simulink model "speedgoat deneme"  (R2015b)
settings: Solver=FixedStepDiscrete  StartTime=0.0  StopTime=inf  RelTol=1e-3
libraries: speedgoatlib_IO102 x4, speedgoatlib_fpga x3, slrtlib x2, simulink x1
settings Model: Creator=PowerLab  LastModifiedBy=PowerLab
settings SolverCC: EnableConcurrentExecution=on
settings OptimizationCC: BlockReduction=off  OptimizeBlockIOStorage=off  BufferReuse=off  GlobalBufferReuse=off  ExpressionFolding=off  LocalBlockOutputs=off
settings HardwareCC: ProdBitPerPointer=32  ProdLargestAtomicFloat=None  ProdWordSize=32  ProdLongLongMode=on  ProdHWDeviceType=Generic->32-bit x86 compatible
settings RTWCC: SystemTargetFile=slrt.tlc  TemplateMakefile=slrt_default_tmf  Description=Simulink Real-Time  RTWCompilerOptimization=on
settings SimulinkRealTimeCC: xPCisModelTimeout=off  xPCModelTimeoutSecs=20

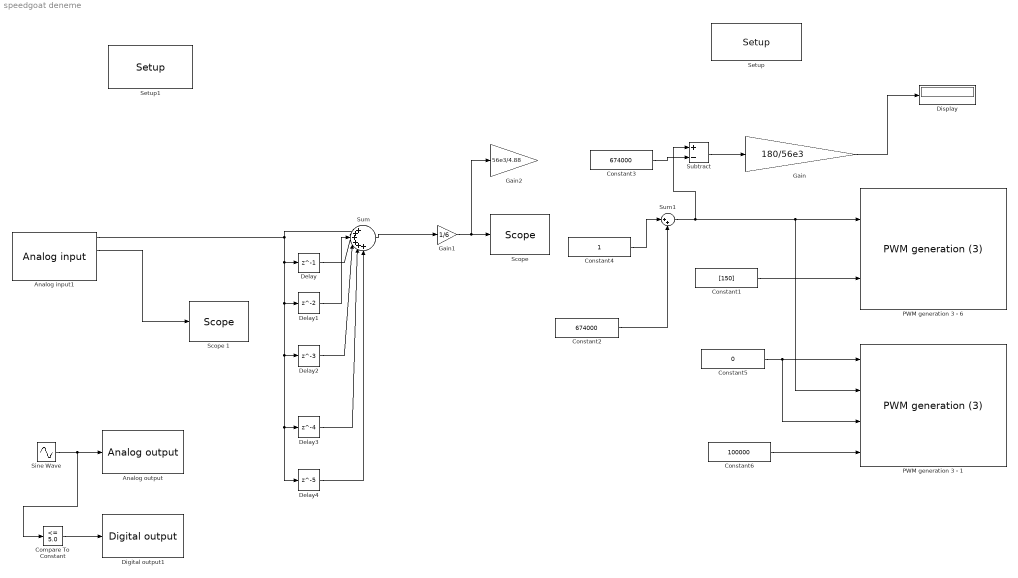
== system speedgoat deneme ==
  Analog input1 : speedgoatlib_IO102/Analog input  id=1  channels=[1,2,3,4]  range=1  high_voltage=off  adCoupling=1  ts=0.001  pciSlot=-1
  Analog output : speedgoatlib_IO102/Analog output  id=1  channels=1  range=1  ts=0.0001  pciSlot=-1
  Compare To Constant : simulink/Logic and Bit Operations/Compare To Constant  relop=<=  const=5.0  OutDataTypeStr=boolean
  Constant1 : Constant  Value=[150]  VectorParams1D=off  OutDataTypeStr=Inherit: Inherit via back propagation
  Constant2 : Constant  Value=674000  VectorParams1D=off  OutDataTypeStr=Inherit: Inherit via back propagation
  Constant3 : Constant  Value=674000  VectorParams1D=off  OutDataTypeStr=Inherit: Inherit via back propagation
  Constant4 : Constant  VectorParams1D=off  OutDataTypeStr=Inherit: Inherit via back propagation
  Constant5 : Constant  Value=0  VectorParams1D=off  OutDataTypeStr=Inherit: Inherit via back propagation
  Constant6 : Constant  Value=100000  VectorParams1D=off  OutDataTypeStr=Inherit: Inherit via back propagation
  Delay : Delay  DelayLength=1
  Delay1 : Delay
  Delay2 : Delay  DelayLength=3
  Delay3 : Delay  DelayLength=4
  Delay4 : Delay  DelayLength=5
  Digital output1 : speedgoatlib_IO102/Digital output  id=1  channels=1  ts=0.001  pciSlot=-1
  Display : Display
  Gain : Gain  Gain=180/56e3
  Gain1 : Gain  Gain=1/6
  Gain2 : Gain  Gain=56e3/4.88
  PWM generation 3 - 1 : speedgoatlib_fpga/PWM/PWM generation (3)  id=1  chan=[1]  board=IO316  ts=0.001  pciSlot=-1  symmetric=Asymmetric - On and Off are freely configurable  period=[1500000]  invertA=High between AOn and AOff  invertB=Low between BOn and BOff  invertC=High during PWM strobe  triggerSource=Period starts  triggerPulseLength=[255]  protection=Disabled: A and B can be high at the same moment  update=At period starts  idleA=Low when PWM generation is halted  idleB=Low when PWM generation is halted
  PWM generation 3 - 6 : speedgoatlib_fpga/PWM/PWM generation (3)  id=1  chan=[3]  board=IO316  ts=0.001  pciSlot=-1  symmetric=Symmetric - PWM generation is centered around half the period  period=[1500000]  invertA=High between AOn and AOff  invertB=High between BOn and BOff  invertC=High during PWM strobe  triggerSource=Period starts  triggerPulseLength=[255]  protection=Disabled: A and B can be high at the same moment  update=At period starts  idleA=Low when PWM generation is halted  idleB=Low when PWM generation is halted
  "Scope " : slrtlib/Displays and Logging/Scope   scopeno=1  scopetype=Target  autostart=on  viewmode=Graphical redraw  formatstr='%15.6f'  grid=on  ylimits=[-10,10]  nosamples=250  noprepostsamples=0  interleave=1  triggermode=FreeRun  triggersignal=1  trigsignalfromport=off  triggerlevel=0.0  triggerslope=Either  triggerscope=1  triggersample=0  filename=data.dat  mode=Lazy  writesize=512  autorestart=off  dynamicfilemode=off  maxwritefilesize=512*1024^2
  Scope 1 : slrtlib/Displays and Logging/Scope   scopeno=2  scopetype=Target  autostart=on  viewmode=Graphical redraw  formatstr='%15.6f'  grid=on  ylimits=[-10,10]  nosamples=250  noprepostsamples=0  interleave=1  triggermode=FreeRun  triggersignal=1  trigsignalfromport=off  triggerlevel=0.0  triggerslope=Either  triggerscope=1  triggersample=0  filename=data.dat  mode=Lazy  writesize=512  autorestart=off  dynamicfilemode=off  maxwritefilesize=512*1024^2
  Setup : speedgoatlib_fpga/Setup/Setup  board=IO316  id=1  frontIO=None  rearIO=None  bitstreamFile=speedgoat_IO316_MotionControl_01325e  ProgSpiFlash=off  ProgBPIFlash=off  pciSlot=-1  PullRPort0=pull-up 3.3V  VioPort0=3.3V  PullRPort1=pull-up 3.3V  VioPort1=3.3V  PullRPort2=pull-up 3.3V  VioPort2=3.3V  PullRPort3=pull-up 3.3V  VioPort3=3.3V  PullRPort4=pull-up 3.3V  VioPort4=3.3V  PullRPort5=pull-up 3.3V  VioPort5=3.3V  PullRPort6=pull-up 3.3V  VioPort6=3.3V  PullRPort15=floating  PullRPort31=pull-up 3.3V  PullRPort47=pull-up 3.3V  PullRPort63=pull-up 3.3V
  Setup1 : speedgoatlib_IO102/Setup  group=Analog input setup  id=1  range=+-10V  cal=off  pciSlot=-1  adChannelMode=Multiple-channel (enter number of channels below)  adChannel=4  adCoupling=Differential  daChannel=[1]  daReset=[1]  daInitValue=[0]  diChannel=[1]  doChannel=[1]  doReset=[1]  doInitValue=[0]
  Sine Wave : Sin  Amplitude=8  Frequency=6280  SampleTime=0
  Subtract : Sum  Inputs=+-
  Sum : Sum  Inputs=|++++++
  Sum1 : Sum  Inputs=|++
  wires:
  Constant1/1 -> PWM generation 3 - 6/2
  Constant3/1 -> Subtract/2
  Subtract/1 -> Gain/1
  Delay/1 -> Sum/2
  Sum/1 -> Gain1/1
  Gain1/1 -> Gain2/1, "Scope "/1
  Delay1/1 -> Sum/3
  Delay2/1 -> Sum/4
  Constant2/1 -> Sum1/2
  Sum1/1 -> Subtract/1, PWM generation 3 - 1/2, PWM generation 3 - 6/1
  Analog input1/1 -> Sum/1, Delay3/1, Delay4/1, Delay2/1, Delay1/1, Delay/1
  Delay3/1 -> Sum/5
  Delay4/1 -> Sum/6
  Gain/1 -> Display/1
  Analog input1/2 -> Scope 1/1
  Constant4/1 -> Sum1/1
  Constant5/1 -> PWM generation 3 - 1/3, PWM generation 3 - 1/1
  Constant6/1 -> PWM generation 3 - 1/4
  Sine Wave/1 -> Compare To Constant/1, Analog output/1
  Compare To Constant/1 -> Digital output1/1
